simulink model "c7mnlrsys"  (Simulink 7.7)
settings: Solver=ode3  StartTime=0.0  StopTime=30000*0.01  FixedStep=0.01  RelTol=1e-3
libraries: simulink x1
settings Model: Creator=Administrator  LastModifiedBy=Professor Dingyu Xue
settings DataIOCC: LimitDataPoints=off
settings OptimizationCC: InitFltsAndDblsToZero=on
settings DebuggingCC: StrictBusMsg=Warning

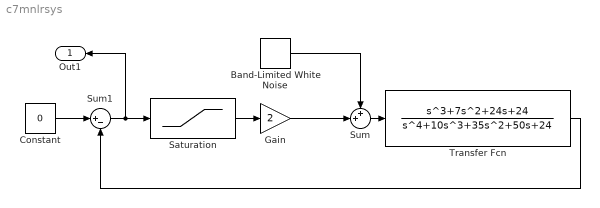
== system c7mnlrsys ==
  Band-Limited White Noise : simulink/Sources/Band-Limited White Noise  SystemSampleTime=-1  Cov=sqrt(3)  Ts=0.01  seed=[23341]
  Constant : Constant  Value=0
  Gain : Gain  Gain=2
  Saturation : Saturate  UpperLimit=1  LowerLimit=-1
  Sum : Sum  Inputs=++|
  Sum1 : Sum  Inputs=|+-
  Transfer Fcn : TransferFcn  Numerator=[1 7 24 24]  Denominator=[1 10 35 50 24]
  Out1 : Outport
  wires:
  Band-Limited White Noise/1 -> Sum/1
  Transfer Fcn/1 -> Sum1/2
  Sum/1 -> Transfer Fcn/1
  Saturation/1 -> Gain/1
  Constant/1 -> Sum1/1
  Sum1/1 -> Saturation/1, Out1/1
  Gain/1 -> Sum/2
